simulink model "swap"  (R2018b)
settings: Solver=VariableStepAuto  StartTime=0.0  StopTime=10.0  RelTol=1e-3
settings Model: Creator=student  LastModifiedBy=pal35

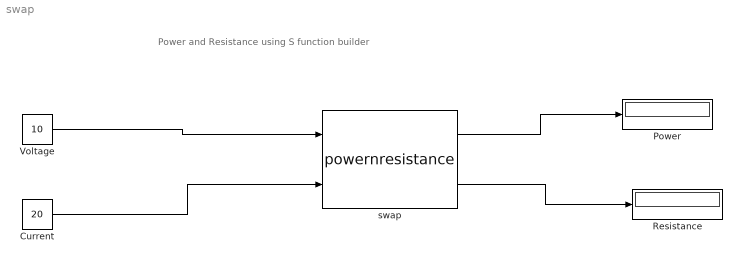
== system swap ==
  note: Power and Resistance using S function builder
  Current : Constant  Value=20
  Power : Display
  Resistance : Display
  Voltage : Constant  Value=10
  swap : S-Function  InitFcn=try, set_param(gcb,'FunctionName','powernresistance'), end  FunctionName=powernresistance  SFunctionModules=powernresistance_wrapper  SFunctionDeploymentMode=off  EnableBusSupport=off  mask(S-Function Builder){}
      mask help: Simulink:masks:SFunctionBuilder_MD
      mask init:
      | val = [[.9  0.75 0.75 1 1 .9 .9 1]',[1 1 0.75 0.75 .9 .9 1 .9]'];try , sys = get_param(gcb,'SfunBuilderFcnName');if isempty(sys), sys = get_param(gcb,'FunctionName'); end,catch, sys = get_param(gcb,'FunctionName'); end
      settings: CopyFcn=set_param(gcbh,'LinkStatus','none')  PreSaveFcn=try, set_param(gcb,'FunctionName','powernresistance'), end  OpenFcn=sfunctionwizard(gcbh)
      mask Display: plot(val(:,1),val(:,2)),disp(sys), port_label('input',1,'voltage'), port_label('input',2,'current'), port_label('output',1,'power'), port_label('output',2,'resistance')
  wires:
  Voltage/1 -> swap/1
  Current/1 -> swap/2
  swap/1 -> Power/1
  swap/2 -> Resistance/1
